simulink model "HWC"  (R2018a)
settings: Solver=FixedStepAuto  StartTime=0.0  StopTime=stopTime  FixedStep=stepSize  RelTol=1e-3
values from neighbouring files (symbols this model uses):
  n = revs_per_day*2*pi/(24*3600)    [TLE_Reader.m]
  rho_RTN_init = T_ECI2RTN*(r2_ECI_init-r_ECI_init)    [AA279D_PSET2.m]    (also in AA279D_PSET2_a_change.m)
  rhod_RTN_init = T_ECI2RTN*(v2_ECI_init-v_ECI_init)-     cross([0;0;thd0],rho_RTN_init)    [AA279D_PSET2.m]    (also in AA279D_PSET2_a_change.m)
  stepSize = 24*60*60/revs_per_day/100000    [AA279D_PSET1.m]    (also in AA279D_PSET2.m = 1; AA279D_PSET2_a_change.m = 5)
settings Model: Creator=Christopher Covert  LastModifiedBy=Christopher Covert

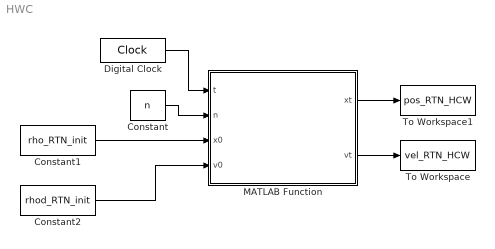
== system HWC ==
  Constant : Constant  Value=n
  Constant1 : Constant  Value=rho_RTN_init
  Constant2 : Constant  Value=rhod_RTN_init
  Digital Clock : DigitalClock  SampleTime=stepSize
  MATLAB Function : MATLAB Function  TreatAsAtomicUnit=on
  To Workspace : ToWorkspace  VariableName=vel_RTN_HCW  SampleTime=-1
  To Workspace1 : ToWorkspace  VariableName=pos_RTN_HCW  SampleTime=-1
  wires:
  Constant/1 -> MATLAB Function/2(n)
  MATLAB Function/1(xt) -> To Workspace1/1
  MATLAB Function/2(vt) -> To Workspace/1
  Constant1/1 -> MATLAB Function/3(x0)
  Constant2/1 -> MATLAB Function/4(v0)
  Digital Clock/1 -> MATLAB Function/1(t)

== matlab function HWC/MATLAB Function ==
  data: t input; n input; xt output; x0 input; v0 input; vt output
function [xt,vt] = HCW_PROP(t,n,x0,v0)

x0 = [x0;v0];

s = sin(n*t);
c = cos(n*t);

eAt = [4-3*c,0,0,s/n,(2/n)-(2*c/n),0;...
    -6*n*t+6*s,1,0,-2/n+2*c/n,4*s/n-3*t,0;...
    0,0,c,0,0,s/n;...
    3*n*s,0,0,c,2*s,0;...
    -6*n+6*n*c,0,0,-2*s,-3+4*c,0;...
    0,0,-n*s,0,0,c];

x = eAt*x0;


xt = x(1:3);
vt = x(4:6);

end
